simulink subsystem "quat_kin_body"  (R2022a)
settings: Solver=VariableStepAuto  StartTime=0.0  StopTime=10.0  RelTol=1e-3
libraries: aerolibutil x1, sharedutil x1
settings Model: Creator=samuel  LastModifiedBy=samuel

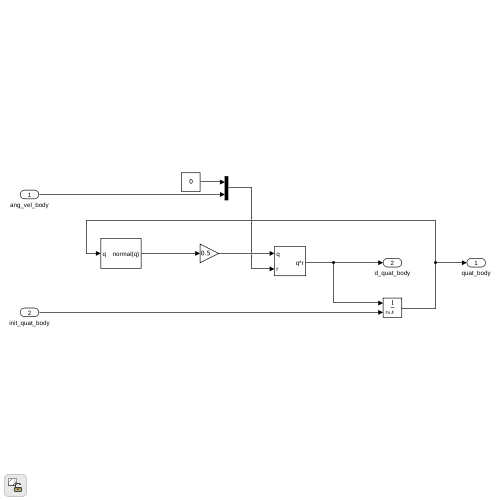
[thumbnail: Simulink's stored preview of the top-level diagram]
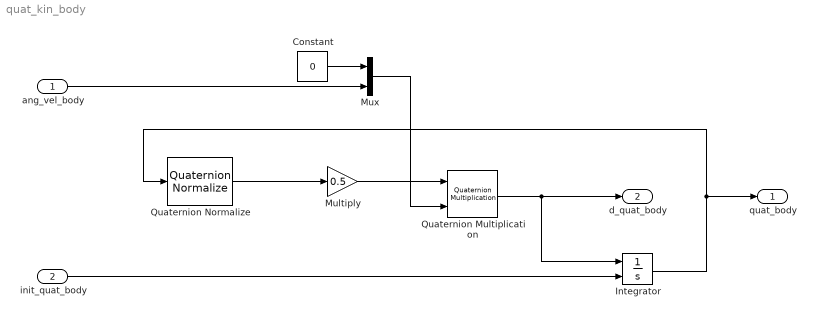
== system quat_kin_body ==
  ang_vel_body : Inport
  init_quat_body : Inport  Port=2
  Constant : Constant  Value=0
  Integrator : Integrator  InitialConditionSource=external
  Multiply : Gain  Gain=0.5
  Mux : Mux  Inputs=2
  Quaternion Multiplication : aerolibutil/Quaternion Multiplication
  Quaternion Normalize : sharedutil/Quaternion Normalize  aMode=aMode
      settings: SourceProductBaseCode=AE,PW,DR,MT,VE
  quat_body : Outport
  d_quat_body : Outport  Port=2
  wires:
  Multiply/1 -> Quaternion Multiplication/1
  Constant/1 -> Mux/1
  ang_vel_body/1 -> Mux/2
  Mux/1 -> Quaternion Multiplication/2
  Quaternion Multiplication/1 -> Integrator/1, d_quat_body/1
  Integrator/1 -> Quaternion Normalize/1, quat_body/1
  Quaternion Normalize/1 -> Multiply/1
  init_quat_body/1 -> Integrator/2
